simulink model "bs_a"  (R2022b)
settings: Solver=ode4  StartTime=0.0  StopTime=10.0  FixedStep=0.01  RelTol=1e-3
libraries: simulink x1
settings Model: Creator=张倬境  LastModifiedBy=张倬境

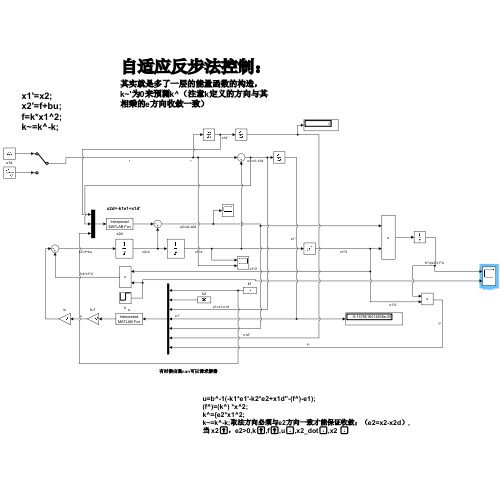
[thumbnail: Simulink's stored preview of the top-level diagram]
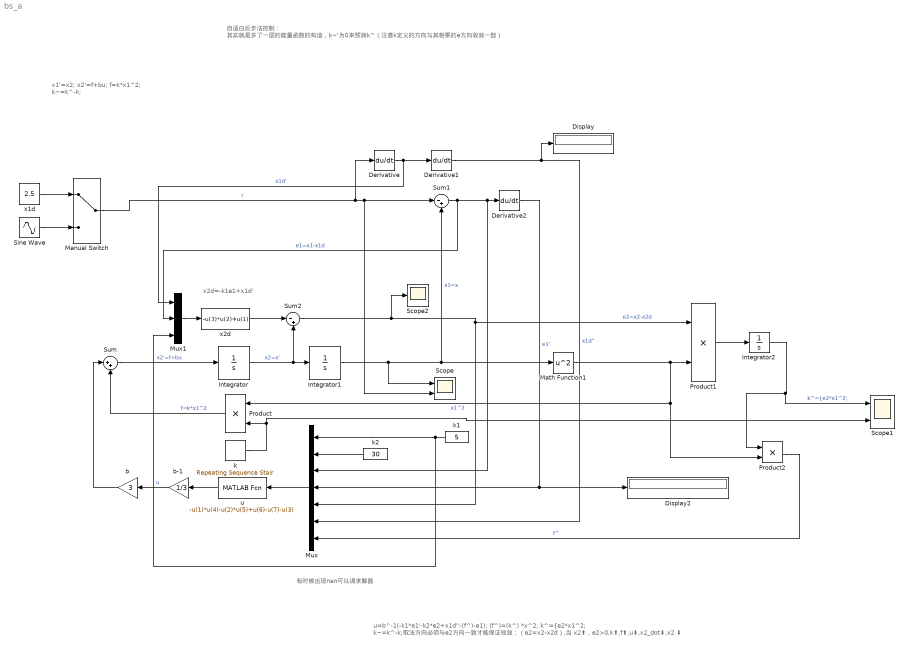
== system bs_a ==
  note: 自适应反步法控制：
      | 其实就是多了一层的能量函数的构造，k~'为0来预测k^（注意k定义的方向与其相乘的e方向收敛一致）
  note: 有时候出现nan可以调求解器
  note: x2d=-k1e1+x1d'
  note: x1'=x2;
      | x2'=f+bu;
      | f=k*x1^2;
      | k~=k^-k;
  note: u=b^-1(-k1*e1'-k2*e2+x1d''-(f^)-e1);
      | (f^)=(k^) *x^2;
      | k^={e2*x1^2;
      | k~=k^-k;取法方向必须与e2方向一致才能保证收敛；（e2=x2-x2d）,当 x2⬆，e2>0,k⬆,f⬆,u⬇,x2_dot⬇,x2 ⬇
  Derivative : Derivative
  Derivative1 : Derivative
  Derivative2 : Derivative
  Display : Display
  Display2 : Display
  Integrator : Integrator
  Integrator1 : Integrator
  Integrator2 : Integrator
  Manual Switch : ManualSwitch
  Math Function1 : Math  Operator=square
  Mux : Mux  Inputs=7
  Mux1 : Mux  Inputs=3
  Product : Product
  Product1 : Product
  Product2 : Product
  Scope : Scope  NumInputPorts=2
  Scope1 : Scope  NumInputPorts=2
  Scope2 : Scope
  Sine Wave : Sin  SampleTime=0
  Sum : Sum  Inputs=|++
  Sum1 : Sum  Inputs=|-+
  Sum2 : Sum  Inputs=|-+
  b : Gain  Gain=3
  b-1 : Gain  Gain=1/3
  k : simulink/Sources/Repeating Sequence Stair  OutValues=[1 2]  tsamp=5  OutMin=[]  OutMax=[]  OutDataTypeStr=double  OutputDataTypeScalingMode=double  OutDataType=fixdt(0,8)  ConRadixGroup=Best Precision: Vector-wise  OutScaling=2^-12
  k1 : Constant  Value=5
  k2 : Constant  Value=30
  u : MATLABFcn  MATLABFcn=-u(1)*u(4)-u(2)*u(5)+u(6)-u(7)-u(3)  OutputDimensions=[1 1]  OutputSignalType=real  Output1D=off
  x1d : Constant  Value=2.5
  x2d : MATLABFcn  MATLABFcn=-u(3)*u(2)+u(1)
  wires:
  Sine Wave/1 -> Manual Switch/2
  Mux/1 -> u/1
  u/1 -> b-1/1
  Derivative2/1 -> Mux/4, Display2/1  "e1'"
  Sum2/1 -> Scope2/1, Mux/5, Product1/1  "e2=x2-x2d"
  Derivative/1 -> Mux1/1, Derivative1/1  "x1d'"
  k2/1 -> Mux/2
  Derivative1/1 -> Display/1, Mux/6  "x1d''"
  x1d/1 -> Manual Switch/1
  Sum1/1 -> Mux1/2, Derivative2/1, Mux/3  "e1=x1-x1d"
  Mux1/1 -> x2d/1
  Sum/1 -> Integrator/1  "x2'=f+bu"
  Product/1 -> Sum/2  "f=k*x1^2"
  b/1 -> Sum/1
  x2d/1 -> Sum2/1
  k1/1 -> Mux1/3, Mux/1
  Integrator1/1 -> Scope/1, Sum1/2, Math Function1/1  "x1=x"
  Manual Switch/1 -> Scope/2, Sum1/1, Derivative/1  "r"
  b-1/1 -> b/1  "u"
  Integrator/1 -> Sum2/2, Integrator1/1  "x2=x'"
  k/1 -> Product/2, Scope1/2
  Product1/1 -> Integrator2/1
  Math Function1/1 -> Product1/2, Product/1, Product2/2  "x1^2"
  Product2/1 -> Mux/7  "f^"
  Integrator2/1 -> Scope1/1, Product2/1  "k^={e2*x1^2;"
